simulink model "CT_CPC_filtro_V75R2010a"  (Simulink 7.5)
settings: Solver=ode45  StartTime=0.0  StopTime=60  FixedStep=Tm  RelTol=1e-3
InitFcn:
  | Tm = 0.01;
libraries: simulink x4
settings Model: Creator=Equipo-Servo  LastModifiedBy=Equipo-Servo  ExtModeTrigDuration=100000
settings OptimizationCC: ExpressionDepthLimit=128
settings DebuggingCC: FcnCallInpInsideContextMsg=Enable All
settings HardwareCC: ProdIntDivRoundTo=Zero  ProdEndianess=LittleEndian  ProdHWDeviceType=Generic->32-bit x86 compatible
settings RTWCC: SystemTargetFile=rtwin.tlc  TemplateMakefile=rtwin.tmf  Description=Real-Time Windows Target  ProcessScript=rtwin_make_rtw_hook  RTWCompilerOptimization=On
settings CodeAppCC: MaxIdLength=95  CustomSymbolStrType=$N$R$M_T
settings RTWinTargetCC: TargetLibSuffix=_rtwin.lib  TargetPreCompLibLocation=C:\Program Files\MATLAB\R2013a\toolbox\rtw\targets\rtwin\lib\win32  TargetFunctionLibrary=ANSI_C  MatFileLogging=on  RTWinDir=C:/PROGRA~1/MATLAB/R2013a/toolbox/rtw/targets/rtwin  TargetArch=win32

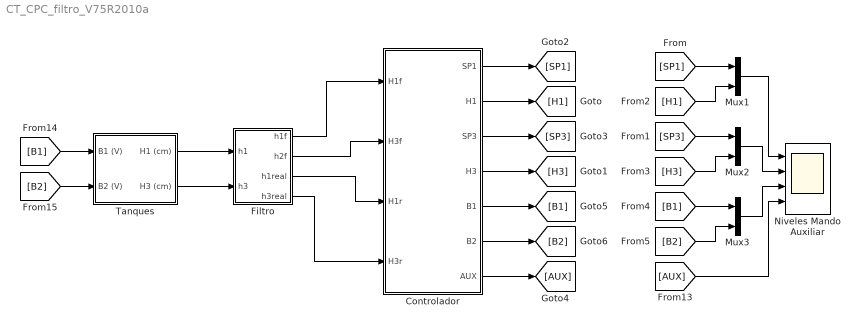
== system CT_CPC_filtro_V75R2010a ==
  Controlador : Subsystem
  Filtro : Subsystem
  Mux1 : Mux  Inputs=2
  Mux2 : Mux  Inputs=2
  Mux3 : Mux  Inputs=2
  Niveles Mando Auxiliar : Scope  NumInputPorts=4
      settings: TimeRange=60  YMin=0~-1~0~-5  YMax=15~1~6~15
  Tanques : Subsystem
  wires:
  Mux1/1 -> Niveles Mando Auxiliar/1
  [SP1] -> Mux1/1
  [H1] -> Mux1/2
  [SP3] -> Mux2/1
  [H3] -> Mux2/2
  Mux2/1 -> Niveles Mando Auxiliar/2
  [B1] -> Mux3/1
  [B2] -> Mux3/2
  Mux3/1 -> Niveles Mando Auxiliar/3
  [AUX] -> Niveles Mando Auxiliar/4
  Controlador/1(SP1) -> [SP1]
  Controlador/2(H1) -> [H1]
  Controlador/3(SP3) -> [SP3]
  Controlador/4(H3) -> [H3]
  Controlador/5(B1) -> [B1]
  Controlador/6(B2) -> [B2]
  Controlador/7(AUX) -> [AUX]
  [B1] -> Tanques/1(B1 (V))
  [B2] -> Tanques/2(B2 (V))
  Filtro/1(h1f) -> Controlador/1(H1f)
  Filtro/2(h2f) -> Controlador/2(H3f)
  Tanques/1(H1 (cm)) -> Filtro/1(h1)
  Tanques/2(H3 (cm)) -> Filtro/2(h3)
  Filtro/3(h1real) -> Controlador/3(H1r)
  Filtro/4(h3real) -> Controlador/4(H3r)

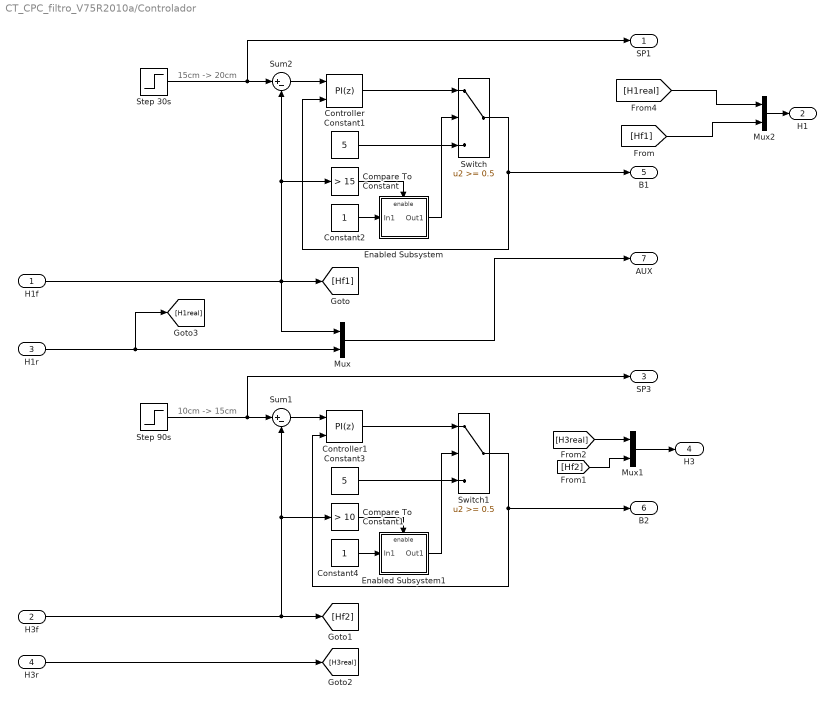
== system CT_CPC_filtro_V75R2010a/Controlador ==
  note: 10cm -> 15cm
  note: 15cm -> 20cm
  H1f : Inport
  H3f : Inport  Port=2
  H1r : Inport  Port=3
  H3r : Inport  Port=4
  Compare To Constant : simulink/Logic and Bit Operations/Compare To Constant  relop=>  const=15  LogicOutDataTypeMode=boolean
  Compare To Constant1 : simulink/Logic and Bit Operations/Compare To Constant  relop=>  const=10  LogicOutDataTypeMode=boolean
  Constant1 : Constant  Value=5
  Constant2 : Constant
  Constant3 : Constant  Value=5
  Constant4 : Constant
  Controller : simulink/Continuous/PID Controller  Controller=PI  TimeDomain=Discrete-time  SampleTime=Tm  IntegratorMethod=Forward Euler  FilterMethod=Forward Euler  Form=Parallel  P=1  I=1  D=0  N=100  InitialConditionSource=internal  InitialConditionForIntegrator=0  InitialConditionForFilter=0  ExternalReset=none  LimitOutput=on  UpperSaturationLimit=5  LowerSaturationLimit=0  LinearizeAsGain=off  AntiWindupMode=back-calculation  Kb=1  TrackingMode=on  Kt=1  PParamMin=[]  PParamMax=[]  IParamMin=[]  IParamMax=[]  DParamMin=[]  DParamMax=[]  NParamMin=[]  NParamMax=[]  KbParamMin=[]  KbParamMax=[]  KtParamMin=[]  KtParamMax=[]  POutMin=[]  POutMax=[]  IOutMin=[]  IOutMax=[]  DOutMin=[]  DOutMax=[]  NOutMin=[]  NOutMax=[]  KbOutMin=[]  KbOutMax=[]  KtOutMin=[]  KtOutMax=[]  IntegratorOutMin=[]  IntegratorOutMax=[]  FilterOutMin=[]  FilterOutMax=[]  SumOutMin=[]  SumOutMax=[]  SumI1OutMin=[]  SumI1OutMax=[]  SumI2OutMin=[]  SumI2OutMax=[]  SumI3OutMin=[]  SumI3OutMax=[]  SumDOutMin=[]  SumDOutMax=[]  SaturationOutMin=[]  SaturationOutMax=[]  IntegratorContinuousStateAttributes=''  IntegratorStateMustResolveToSignalObject=off  IntegratorRTWStateStorageClass=Auto  FilterContinuousStateAttributes=''  FilterStateMustResolveToSignalObject=off  FilterRTWStateStorageClass=Auto
  Controller1 : simulink/Continuous/PID Controller  Controller=PI  TimeDomain=Discrete-time  SampleTime=Tm  IntegratorMethod=Forward Euler  FilterMethod=Forward Euler  Form=Parallel  P=1  I=1  D=0  N=100  InitialConditionSource=internal  InitialConditionForIntegrator=0  InitialConditionForFilter=0  ExternalReset=none  LimitOutput=on  UpperSaturationLimit=5  LowerSaturationLimit=0  LinearizeAsGain=off  AntiWindupMode=back-calculation  Kb=1  TrackingMode=on  Kt=1  PParamMin=[]  PParamMax=[]  IParamMin=[]  IParamMax=[]  DParamMin=[]  DParamMax=[]  NParamMin=[]  NParamMax=[]  KbParamMin=[]  KbParamMax=[]  KtParamMin=[]  KtParamMax=[]  POutMin=[]  POutMax=[]  IOutMin=[]  IOutMax=[]  DOutMin=[]  DOutMax=[]  NOutMin=[]  NOutMax=[]  KbOutMin=[]  KbOutMax=[]  KtOutMin=[]  KtOutMax=[]  IntegratorOutMin=[]  IntegratorOutMax=[]  FilterOutMin=[]  FilterOutMax=[]  SumOutMin=[]  SumOutMax=[]  SumI1OutMin=[]  SumI1OutMax=[]  SumI2OutMin=[]  SumI2OutMax=[]  SumI3OutMin=[]  SumI3OutMax=[]  SumDOutMin=[]  SumDOutMax=[]  SaturationOutMin=[]  SaturationOutMax=[]  IntegratorContinuousStateAttributes=''  IntegratorStateMustResolveToSignalObject=off  IntegratorRTWStateStorageClass=Auto  FilterContinuousStateAttributes=''  FilterStateMustResolveToSignalObject=off  FilterRTWStateStorageClass=Auto
  Enabled Subsystem : Subsystem  TreatAsAtomicUnit=on
  Enabled Subsystem1 : Subsystem  TreatAsAtomicUnit=on
  Mux : Mux  Inputs=2
  Mux1 : Mux  Inputs=2
  Mux2 : Mux  Inputs=2
  Step 30s : Step  Time=40  Before=15  After=25  SampleTime=0
  Step 90s : Step  Time=90  Before=10  After=15  SampleTime=0
  Sum1 : Sum  Inputs=|+-
  Sum2 : Sum  Inputs=|+-
  Switch : Switch  Threshold=0.5
  Switch1 : Switch  Threshold=0.5
  SP1 : Outport
  H1 : Outport  Port=2
  SP3 : Outport  Port=3
  H3 : Outport  Port=4
  B1 : Outport  Port=5
  B2 : Outport  Port=6
  AUX : Outport  Port=7
  wires:
  Enabled Subsystem1/1(Out1) -> Switch1/2
  Switch1/1 -> Controller1/2, B2/1
  Sum1/1 -> Controller1/1
  Constant4/1 -> Enabled Subsystem1/1(In1)
  Compare To Constant1/1 -> Enabled Subsystem1/Enable
  Constant3/1 -> Switch1/3
  Controller1/1 -> Switch1/1
  H3f/1 -> [Hf2], Compare To Constant1/1, Sum1/2
  Step 90s/1 -> Sum1/1, SP3/1
  Enabled Subsystem/1(Out1) -> Switch/2
  Switch/1 -> B1/1, Controller/2
  Sum2/1 -> Controller/1
  Constant2/1 -> Enabled Subsystem/1(In1)
  Compare To Constant/1 -> Enabled Subsystem/Enable
  Constant1/1 -> Switch/3
  Controller/1 -> Switch/1
  Mux/1 -> AUX/1
  H1f/1 -> Sum2/2, Compare To Constant/1, Mux/1, [Hf1]
  Step 30s/1 -> Sum2/1, SP1/1
  H1r/1 -> [H1real], Mux/2
  H3r/1 -> [H3real]
  Mux1/1 -> H3/1
  Mux2/1 -> H1/1
  [H3real] -> Mux1/1
  [Hf2] -> Mux1/2
  [H1real] -> Mux2/1
  [Hf1] -> Mux2/2

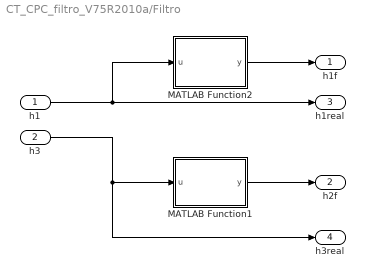
== system CT_CPC_filtro_V75R2010a/Filtro ==
  h1 : Inport
  h3 : Inport  Port=2
  MATLAB Function1 : Stateflow chart  TreatAsAtomicUnit=on
      settings: PermitHierarchicalResolution=ParametersOnly
  MATLAB Function2 : Stateflow chart  TreatAsAtomicUnit=on
      settings: PermitHierarchicalResolution=ParametersOnly
  h1f : Outport
  h2f : Outport  Port=2
  h1real : Outport  Port=3
  h3real : Outport  Port=4
  wires:
  h3/1 -> MATLAB Function1/1(u), h3real/1
  h1/1 -> h1real/1, MATLAB Function2/1(u)
  MATLAB Function1/1(y) -> h2f/1
  MATLAB Function2/1(y) -> h1f/1

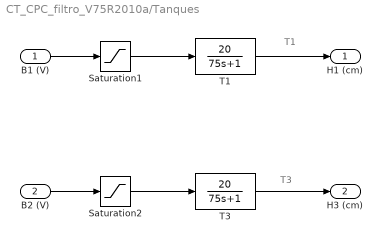
== system CT_CPC_filtro_V75R2010a/Tanques ==
  note: T3
  note: T1
  B1 (V) : Inport
  B2 (V) : Inport  Port=2
  Saturation1 : Saturate  UpperLimit=5  LowerLimit=0
  Saturation2 : Saturate  UpperLimit=5  LowerLimit=0
  T1 : TransferFcn  Numerator=[20]  Denominator=[75 1]
  T3 : TransferFcn  Numerator=[20]  Denominator=[75 1]
  H1 (cm) : Outport
  H3 (cm) : Outport  Port=2
  wires:
  T1/1 -> H1 (cm)/1
  B1 (V)/1 -> Saturation1/1
  Saturation1/1 -> T1/1
  B2 (V)/1 -> Saturation2/1
  Saturation2/1 -> T3/1
  T3/1 -> H3 (cm)/1

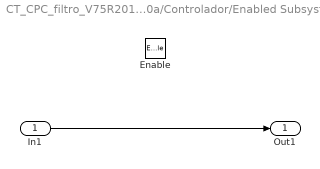
== system CT_CPC_filtro_V75R2010a/Controlador/Enabled Subsystem ==
  In1 : Inport
  Enable : EnablePort
  Out1 : Outport
  wires:
  In1/1 -> Out1/1

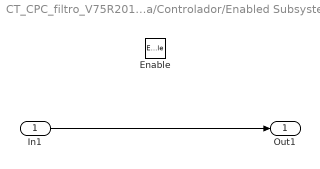
== system CT_CPC_filtro_V75R2010a/Controlador/Enabled Subsystem1 ==
  In1 : Inport
  Enable : EnablePort
  Out1 : Outport
  wires:
  In1/1 -> Out1/1

== matlab function Filtro/MATLAB Function1 ==
  data: u input double; y output double
function y = fcn(u)
%#eml
Tm = 0.5;
alpha = exp(-1*Tm);
persistent yk
if isempty(yk)
    yk = 0;
end

yk = alpha*yk + (1 - alpha)*u;

y = yk;

== matlab function Filtro/MATLAB Function2 ==
  data: u input double; y output double
function y = fcn(u)
%#eml
Tm = 0.5;
alpha = exp(-1*Tm);
persistent yk
if isempty(yk)
    yk = 0;
end

%% filtro de primer orden
yk = alpha*yk + (1 - alpha)*u;

y = yk;
